simulink model "Assem_PhaseI_Ver5"  (R2025a)
settings: Solver=ode45  StartTime=0.0  StopTime=3  MaxStep=0.01  RelTol=1e-3
values from neighbouring files (symbols this model uses):
  Inner = [14.14 0.013 100]    [Assem_PhaseI_Ver5_DataFile.m]
  Ke = 1.215224811858674    (= 1.21522481186)    [Assem_PhaseI_Ver5_DataFile.m]
  Km = 2.170880419565582    (= 2.17088041957)    [Assem_PhaseI_Ver5_DataFile.m]
  Lm = 5.574912164379065e-04    (= 0.000557491216438)    [Assem_PhaseI_Ver5_DataFile.m]
  Outer = [13.249 3.059]    [Assem_PhaseI_Ver5_DataFile.m]
  Rm = 12.324873118212627    (= 12.3248731182)    [Assem_PhaseI_Ver5_DataFile.m]
undefined symbols (not defined in the file or in its folder): _body_Default_sldprt, _Default_sldprt, _fr_Default_sldprt, CL, HFZ20, Kd_pos, Ki_vel, N_pos, smiData, X, Y, Z
libraries: sm_lib x194, nesl_utility x6, simulink_extras x4, slpidlib x2, shareduavrstlib x1
(part 1 of 5)
settings Model: Creator=rajap  LastModifiedBy=rajap
settings DataIOCC: ExternalInput=[Damping, Rod_Damping]

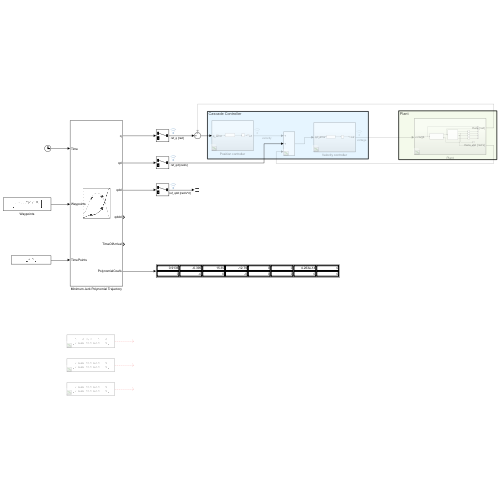
[thumbnail: Simulink's stored preview of the top-level diagram]
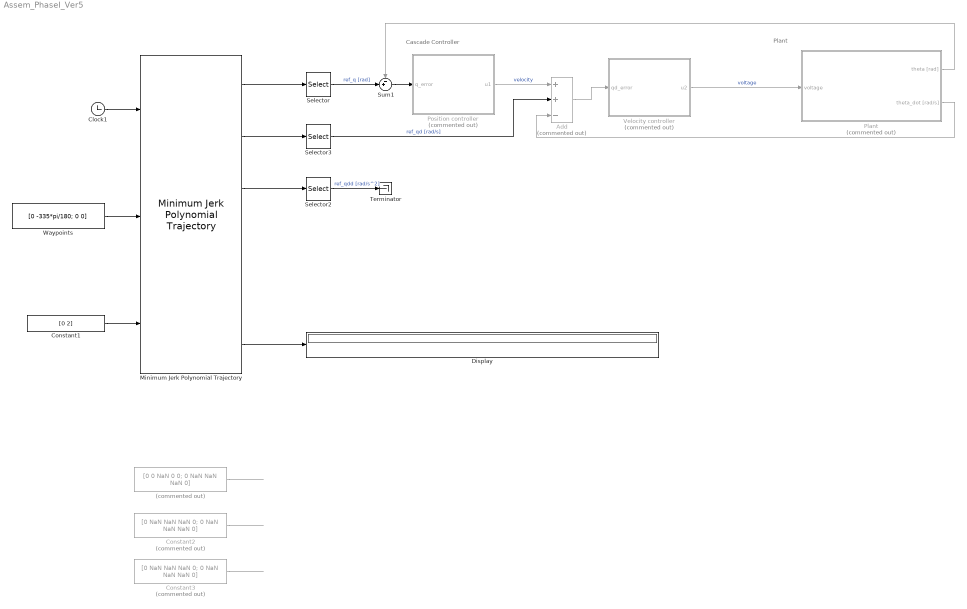
== system Assem_PhaseI_Ver5 ==
  note: Plant
  note: Cascade Controller
  " " : Constant  Commented=on  Value=[0 0 NaN 0 0; 0 NaN NaN NaN 0]
  Add : Sum  Commented=on  Inputs=++-
  Clock1 : Clock
  Constant1 : Constant  Value=[0 2]
  Constant2 : Constant  Commented=on  Value=[0 NaN NaN NaN 0; 0 NaN NaN NaN 0]
  Constant3 : Constant  Commented=on  Value=[0 NaN NaN NaN 0; 0 NaN NaN NaN 0]
  Display : Display
  Minimum Jerk Polynomial Trajectory : shareduavrstlib/Minimum Jerk Polynomial Trajectory  ShowBCInputPort=off  ShowPolynomialCoefs=on  ShowStatusOutputPort=off  TimeAllocation=off  TimeWeight=100  MinSegmentTime=0.1  MaxSegmentTime=1  MaxIteration=1500  MaxTime=10  SimulateUsing=Interpreted execution
      settings: LibrarySourceBlock=robotutilslib/Minimum Jerk Polynomial Trajectory
  Plant : Subsystem  Commented=on
  Position controller : Subsystem  Commented=on
  Selector : Selector  InputPortWidth=2  IndexOptions=Index vector (dialog)  Indices=[1]  OutputSizes=1
  Selector2 : Selector  InputPortWidth=2  IndexOptions=Index vector (dialog)  Indices=[1]  OutputSizes=1
  Selector3 : Selector  InputPortWidth=2  IndexOptions=Index vector (dialog)  Indices=[1]  OutputSizes=1
  Sum1 : Sum  Inputs=-+|
  Terminator : Terminator
  Velocity controller : Subsystem  Commented=on
  Waypoints : Constant  Value=[0 -335*pi/180; 0 0]
  wires:
  Position controller/1(u1) -> Add/1  "velocity"
  Sum1/1 -> Position controller/1(q_error)
  Add/1 -> Velocity controller/1(qd_error)
  Plant/1(theta [rad]) -> Sum1/1
  Clock1/1 -> Minimum Jerk Polynomial Trajectory/1
  Waypoints/1 -> Minimum Jerk Polynomial Trajectory/2
  Constant1/1 -> Minimum Jerk Polynomial Trajectory/3
  Minimum Jerk Polynomial Trajectory/1 -> Selector/1
  Minimum Jerk Polynomial Trajectory/2 -> Selector3/1
  Selector3/1 -> Add/2  "ref_qd [rad/s]"
  Selector/1 -> Sum1/2  "ref_q [rad]"
  Minimum Jerk Polynomial Trajectory/6 -> Display/1
  Minimum Jerk Polynomial Trajectory/3 -> Selector2/1
  Selector2/1 -> Terminator/1  "ref_qdd [rad/s^2]"
  " "/1 -> ?
  Constant2/1 -> ?
  Constant3/1 -> ?
  Velocity controller/1(u2) -> Plant/1(voltage)  "voltage"
  Plant/2(theta_dot [rad/s]) -> Add/3

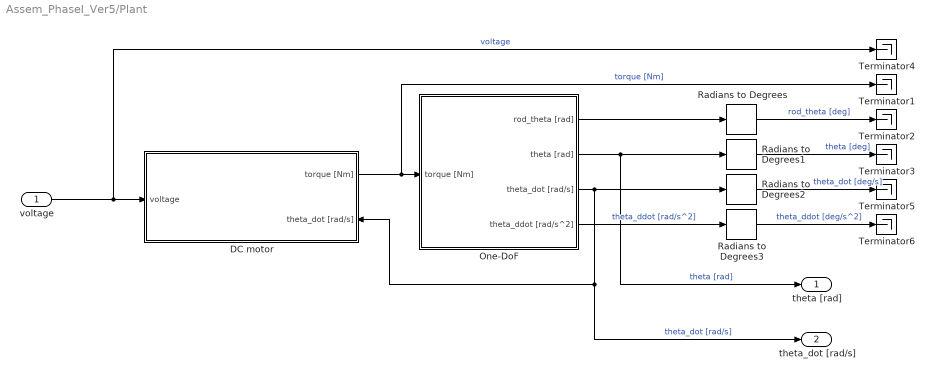
== system Assem_PhaseI_Ver5/Plant ==
  voltage : Inport
  DC motor : Subsystem
      settings: PortSchema="{\"entries\":[{\"content\":{\"sides\":[{\"content\":{\"connectorIds\":[\"In1\"]},\"type\":\"ConnectorPlacement.EquallySpacedRectSide\",\"uuid\":\"4f86a9b4-d250-4a00-a21b-7a5039b64f0e\"},{\"content\":{\"connectorIds\":[\"Out1\",\"In2\"],\"side\":\"RIGHT\"},\"type\":\"ConnectorPlacement.EquallySpacedRectSide\",\"uuid\":\"0247b462-0adc-43ca-ab8f-41e608c3493f\"},{\"content\":{\"side\":\"TOP\"},\"type\":\"ConnectorPlacement.EquallySpacedRectSide\",\"uuid\":\"421294b6-0877-49d2-b28f-df3315123750\"}]},\"type\":\"ConnectorPlacement.EquallySpacedConnector\",\"uuid\":\"bbd11727-88d6-4b17-aa5c-d83762864dc5\"}],\"packageUris\":[\"http://schema.mathworks.com/mf0/Connector/R2020b\"],\"version\":\"1.0\"}"
  One-DoF : Subsystem  InitFcn=run('Assem_PhaseI_Ver5_DataFile.m');
  Radians to Degrees{,1..3} (4 alike) : simulink_extras/Transformations/Radians to Degrees
  Terminator{1..6} (6 alike) : Terminator
  theta [rad] : Outport
  theta_dot [rad/s] : Outport  Port=2
  wires:
  One-DoF/3(theta_dot [rad/s]) -> Radians to Degrees2/1, theta_dot [rad/s]/1, DC motor/2(theta_dot [rad/s])  "theta_dot [rad/s]"
  Radians to Degrees3/1 -> Terminator6/1  "theta_ddot [deg/s^2]"
  Radians to Degrees2/1 -> Terminator5/1  "theta_dot [deg/s]"
  Radians to Degrees/1 -> Terminator2/1  "rod_theta [deg]"
  DC motor/1(torque [Nm]) -> Terminator1/1, One-DoF/1(torque [Nm])  "torque [Nm]"
  One-DoF/2(theta [rad]) -> theta [rad]/1, Radians to Degrees1/1  "theta [rad]"
  One-DoF/4(theta_ddot [rad/s^2]) -> Radians to Degrees3/1  "theta_ddot [rad/s^2]"
  voltage/1 -> Terminator4/1, DC motor/1(voltage)  "voltage"
  Radians to Degrees1/1 -> Terminator3/1  "theta [deg]"
  One-DoF/1(rod_theta [rad]) -> Radians to Degrees/1

== system Assem_PhaseI_Ver5/Position controller ==
  q_error : Inport
  Controller Sampling : RateTransition  OutPortSampleTime=0.01
  PID Controller4 : slpidlib/PID Controller  Controller=PI  Form=Parallel  TimeDomain=Continuous-time  UseExternalTs=off  SampleTime=-1  IntegratorMethod=Forward Euler  FilterMethod=Forward Euler  ControllerParametersSource=internal  P=Outer(1)  I=Outer(2)  UseKiTs=off  D=Kd_pos  UseExternalDerivativeSource=off  N=N_pos  UseFilter=on  TunerSelectOption=Transfer Function Based (PID Tuner App)  InitialConditionSource=internal  InitialConditionForIntegrator=0  InitialConditionForFilter=0  DifferentiatorICPrevScaledInput=0  ExternalReset=none  TrackingMode=off  Kt=1  LimitOutput=on  SatLimitsSource=internal  UpperSaturationLimit=5.31  LowerSaturationLimit=-5.31  LinearizeAsGain=on  AntiWindupMode=clamping  Kb=1  LimitIntegrator=off  UpperIntegratorSaturationLimit=inf  LowerIntegratorSaturationLimit=-inf  POutMin=[]  POutMax=[]  IOutMin=[]  IOutMax=[]  DOutMin=[]  DOutMax=[]  NOutMin=[]  NOutMax=[]  SumOutMin=[]  SumOutMax=[]  SaturationOutMin=[]  SaturationOutMax=[]  PParamMin=[]  PParamMax=[]  IParamMin=[]  IParamMax=[]  DParamMin=[]  DParamMax=[]  NParamMin=[]  NParamMax=[]  KbParamMin=[]  KbParamMax=[]  KtParamMin=[]  KtParamMax=[]  KbOutMin=[]  KbOutMax=[]  KtOutMin=[]  KtOutMax=[]  IntegratorOutMin=[]  IntegratorOutMax=[]  FilterOutMin=[]  FilterOutMax=[]  SumI1OutMin=[]  SumI1OutMax=[]  SumI2OutMin=[]  SumI2OutMax=[]  SumI3OutMin=[]  SumI3OutMax=[]  SumI4OutMin=[]  SumI4OutMax=[]  SumDOutMin=[]  SumDOutMax=[]  DifferentiatorOutMin=[]  DifferentiatorOutMax=[]  FilterDiffOutCoefMin=[]  FilterDiffOutCoefMax=[]  ReciprocalOutMin=[]  ReciprocalOutMax=[]  SumDenOutMin=[]  SumDenOutMax=[]  SumNumOutMin=[]  SumNumOutMax=[]  DivideOutMin=[]  DivideOutMax=[]  UdiffTsProdOutMin=[]  UdiffTsProdOutMax=[]  NTsProdOutMin=[]  NTsProdOutMax=[]  UintegralTsProdOutMin=[]  UintegralTsProdOutMax=[]  UngainTsProdOutMin=[]  UngainTsProdOutMax=[]  ClampingZeroOutDataTypeStr=Inherit: Inherit via back propagation  ClampingZeroOutMin=[]  ClampingZeroOutMax=[]  FilterDenConstantOutDataTypeStr=Inherit: Inherit via back propagation  FilterDenConstantOutMin=[]  FilterDenConstantOutMax=[]  PCopyOutDataTypeStr=Inherit: Inherit via back propagation  PCopyOutMin=[]  PCopyOutMax=[]  NCopyOutDataTypeStr=Inherit: Inherit via back propagation  NCopyOutMin=[]  NCopyOutMax=[]  IntegratorContinuousStateAttributes=''  IntegratorStateMustResolveToSignalObject=off  IntegratorRTWStateStorageClass=Auto  FilterContinuousStateAttributes=''  FilterStateMustResolveToSignalObject=off  FilterRTWStateStorageClass=Auto  ParallelPVariant=InternalParameters  IdealPVariant=Disabled  IVariant=InternalParameters  DVariant=Disabled  IntegratorVariant=Continuous  SatVariant=Enabled  AWVariant=ContClampingParallel  PCopyVariant=Disabled  TRVariant=Disabled  FdbkBlocksVariant=Forward  IdealPFdbkVariant=Disabled  SatFdbkVariant=Disabled  DerivativeFilterVariant=Disabled  NVariant=Disabled  NCopyVariant=Disabled_SignalSpec  FilterICVariant=Disabled  IntegratorICVariant=InternalICs  ExternalResetVariant=Disabled  TRSumVariant=Passthrough  SumFdbkVariant=Disabled  SumVariant=Sum_PI  TsampFilterVariant=InternalTs  TsampNgainVariant=Passthrough  TsampIntegralVariant=Disabled_SignalSpec  ExternalSaturationOutDataTypeStr=Inherit: Same as second input  DerivativeSourceVariant=Disabled  PreIntVariant=InternalPreInt
  u1 : Outport
  wires:
  Controller Sampling/1 -> u1/1
  q_error/1 -> PID Controller4/1
  PID Controller4/1 -> Controller Sampling/1

== system Assem_PhaseI_Ver5/Velocity controller ==
  qd_error : Inport
  Controller Sampling : RateTransition  OutPortSampleTime=0.005
  PID Controller4 : slpidlib/PID Controller  Controller=PD  Form=Parallel  TimeDomain=Continuous-time  UseExternalTs=off  SampleTime=-1  IntegratorMethod=Forward Euler  FilterMethod=Forward Euler  ControllerParametersSource=internal  P=Inner(1)  I=Ki_vel  UseKiTs=off  D=Inner(2)  UseExternalDerivativeSource=off  N=Inner(3)  UseFilter=on  TunerSelectOption=Transfer Function Based (PID Tuner App)  InitialConditionSource=internal  InitialConditionForIntegrator=0  InitialConditionForFilter=0  DifferentiatorICPrevScaledInput=0  ExternalReset=none  TrackingMode=off  Kt=1  LimitOutput=on  SatLimitsSource=internal  UpperSaturationLimit=24  LowerSaturationLimit=-24  LinearizeAsGain=on  AntiWindupMode=clamping  Kb=1  LimitIntegrator=off  UpperIntegratorSaturationLimit=inf  LowerIntegratorSaturationLimit=-inf  POutMin=[]  POutMax=[]  IOutMin=[]  IOutMax=[]  DOutMin=[]  DOutMax=[]  NOutMin=[]  NOutMax=[]  SumOutMin=[]  SumOutMax=[]  SaturationOutMin=[]  SaturationOutMax=[]  PParamMin=[]  PParamMax=[]  IParamMin=[]  IParamMax=[]  DParamMin=[]  DParamMax=[]  NParamMin=[]  NParamMax=[]  KbParamMin=[]  KbParamMax=[]  KtParamMin=[]  KtParamMax=[]  KbOutMin=[]  KbOutMax=[]  KtOutMin=[]  KtOutMax=[]  IntegratorOutMin=[]  IntegratorOutMax=[]  FilterOutMin=[]  FilterOutMax=[]  SumI1OutMin=[]  SumI1OutMax=[]  SumI2OutMin=[]  SumI2OutMax=[]  SumI3OutMin=[]  SumI3OutMax=[]  SumI4OutMin=[]  SumI4OutMax=[]  SumDOutMin=[]  SumDOutMax=[]  DifferentiatorOutMin=[]  DifferentiatorOutMax=[]  FilterDiffOutCoefMin=[]  FilterDiffOutCoefMax=[]  ReciprocalOutMin=[]  ReciprocalOutMax=[]  SumDenOutMin=[]  SumDenOutMax=[]  SumNumOutMin=[]  SumNumOutMax=[]  DivideOutMin=[]  DivideOutMax=[]  UdiffTsProdOutMin=[]  UdiffTsProdOutMax=[]  NTsProdOutMin=[]  NTsProdOutMax=[]  UintegralTsProdOutMin=[]  UintegralTsProdOutMax=[]  UngainTsProdOutMin=[]  UngainTsProdOutMax=[]  ClampingZeroOutDataTypeStr=Inherit: Inherit via back propagation  ClampingZeroOutMin=[]  ClampingZeroOutMax=[]  FilterDenConstantOutDataTypeStr=Inherit: Inherit via back propagation  FilterDenConstantOutMin=[]  FilterDenConstantOutMax=[]  PCopyOutDataTypeStr=Inherit: Inherit via back propagation  PCopyOutMin=[]  PCopyOutMax=[]  NCopyOutDataTypeStr=Inherit: Inherit via back propagation  NCopyOutMin=[]  NCopyOutMax=[]  IntegratorContinuousStateAttributes=''  IntegratorStateMustResolveToSignalObject=off  IntegratorRTWStateStorageClass=Auto  FilterContinuousStateAttributes=''  FilterStateMustResolveToSignalObject=off  FilterRTWStateStorageClass=Auto  ParallelPVariant=InternalParameters  IdealPVariant=Disabled  IVariant=Disabled  DVariant=InternalParameters  IntegratorVariant=Disabled  SatVariant=Enabled  AWVariant=Disabled  PCopyVariant=Disabled  TRVariant=Disabled  FdbkBlocksVariant=Forward  IdealPFdbkVariant=Disabled  SatFdbkVariant=Disabled  DerivativeFilterVariant=ContFilter  NVariant=InternalParameters  NCopyVariant=Disabled  FilterICVariant=InternalICsFilter  IntegratorICVariant=Disabled  ExternalResetVariant=Disabled  TRSumVariant=Passthrough  SumFdbkVariant=Disabled  SumVariant=Sum_PD  TsampFilterVariant=InternalTs  TsampNgainVariant=Passthrough  TsampIntegralVariant=Disabled_SignalSpec  ExternalSaturationOutDataTypeStr=Inherit: Same as second input  DerivativeSourceVariant=ErrorSignal  PreIntVariant=InternalPreInt
  u2 : Outport
  wires:
  Controller Sampling/1 -> u2/1
  PID Controller4/1 -> Controller Sampling/1  "v_pid"
  qd_error/1 -> PID Controller4/1

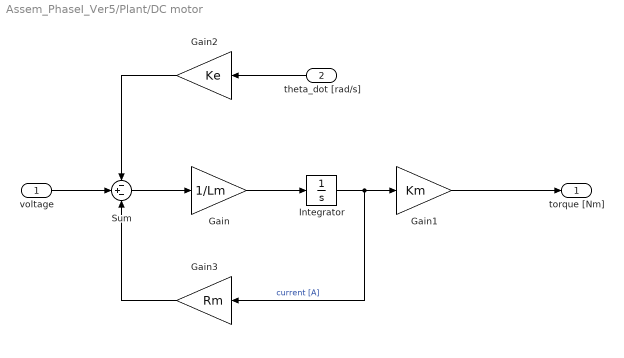
== system Assem_PhaseI_Ver5/Plant/DC motor ==
  voltage : Inport
  theta_dot [rad/s] : Inport  Port=2
  Gain : Gain  Gain=1/Lm
  Gain1 : Gain  Gain=Km
  Gain2 : Gain  Gain=Ke
  Gain3 : Gain  Gain=Rm
  Integrator : Integrator
  Sum : Sum  Inputs=-+-
  torque [Nm] : Outport
  wires:
  voltage/1 -> Sum/2
  Sum/1 -> Gain/1
  Gain3/1 -> Sum/3
  Gain2/1 -> Sum/1
  Integrator/1 -> Gain1/1, Gain3/1  "current [A]"
  Gain/1 -> Integrator/1
  Gain1/1 -> torque [Nm]/1
  theta_dot [rad/s]/1 -> Gain2/1
